simulink model "Part1_3"  (R2020a)
settings: Solver=VariableStepAuto  StartTime=0.0  StopTime=200  RelTol=1e-3
values from neighbouring files (symbols this model uses):
  b = 50    [Script1.m]
  m = 1000    [Script1.m]
  V = 90    [Script1.m]
libraries: cstblocks x1
settings Model: Creator=maxen  LastModifiedBy=maxen

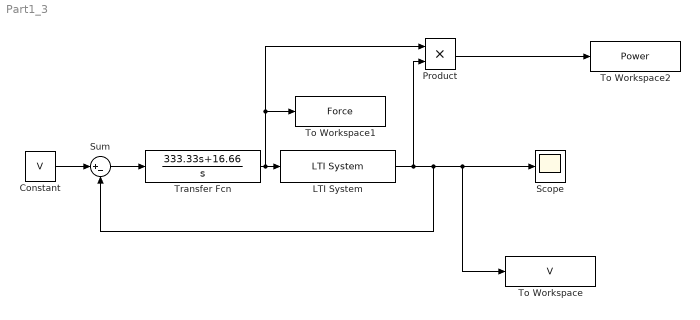
== system Part1_3 ==
  Constant : Constant  Value=V
  LTI System : cstblocks/LTI System  sys=tf(1,[m b])  IC=[]
  Product : Product
  Scope : Scope
  Sum : Sum  Inputs=|+-
  To Workspace : ToWorkspace  VariableName=V  SampleTime=-1
  To Workspace1 : ToWorkspace  VariableName=Force  SampleTime=-1
  To Workspace2 : ToWorkspace  VariableName=Power  SampleTime=-1
  Transfer Fcn : TransferFcn  Numerator=[333.33 16.66]  Denominator=[1 0]
  wires:
  LTI System/1 -> Product/2, To Workspace/1, Scope/1, Sum/2
  Transfer Fcn/1 -> Product/1, To Workspace1/1, LTI System/1
  Constant/1 -> Sum/1
  Sum/1 -> Transfer Fcn/1
  Product/1 -> To Workspace2/1
